simulink model "ps3_1"  (R2020a)
settings: Solver=VariableStepAuto  StartTime=0.0  StopTime=2  RelTol=1e-3
undefined symbols (not defined in the file or in its folder): j
settings Model: Creator=dinhm  LastModifiedBy=dinhm

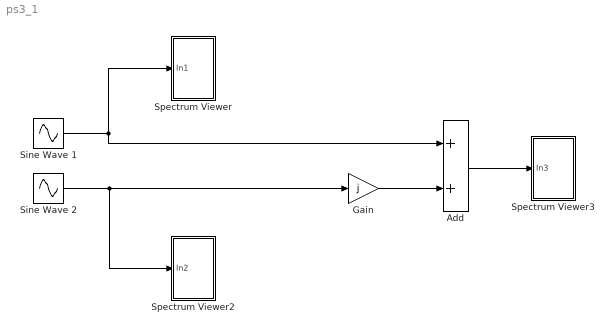
== system ps3_1 ==
  Add : Sum
  Gain : Gain  Gain=j
  Sine Wave 1 : Sin  Frequency=21000  Phase=pi/2  SampleTime=0
  Sine Wave 2 : Sin  Frequency=2*pi*3e3  Phase=78  SampleTime=0
  Spectrum Viewer : Subsystem
  Spectrum Viewer2 : Subsystem
  Spectrum Viewer3 : Subsystem
  wires:
  Sine Wave 2/1 -> Gain/1, Spectrum Viewer2/1(In2)
  Gain/1 -> Add/2
  Sine Wave 1/1 -> Spectrum Viewer/1(In1), Add/1
  Add/1 -> Spectrum Viewer3/1(In3)

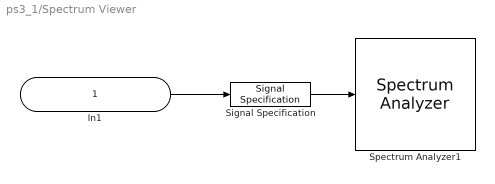
== system ps3_1/Spectrum Viewer ==
  In1 : Inport  Description=In1
  Signal Specification : SignalSpecification  SampleTime=1/16e4
  Spectrum Analyzer1 : SpectrumAnalyzer
  wires:
  Signal Specification/1 -> Spectrum Analyzer1/1
  In1/1 -> Signal Specification/1

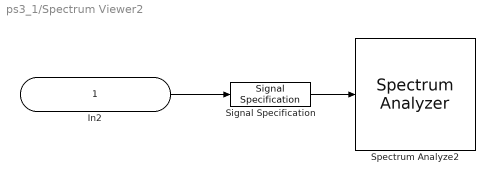
== system ps3_1/Spectrum Viewer2 ==
  In2 : Inport  Description=In1
  Signal Specification : SignalSpecification  SampleTime=1/16e4
  Spectrum Analyze2 : SpectrumAnalyzer
  wires:
  Signal Specification/1 -> Spectrum Analyze2/1
  In2/1 -> Signal Specification/1

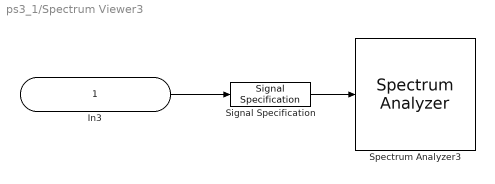
== system ps3_1/Spectrum Viewer3 ==
  In3 : Inport  Description=In1
  Signal Specification : SignalSpecification  SampleTime=1/16e4
  Spectrum Analyzer3 : SpectrumAnalyzer
  wires:
  Signal Specification/1 -> Spectrum Analyzer3/1
  In3/1 -> Signal Specification/1
